simulink subsystem "EncoderAdryvelZ"  (R2023b)
settings: Solver=VariableStepAuto  StartTime=0.0  StopTime=10.0  RelTol=1e-3
libraries: arduinosensorlib x2, simulink x1
settings Model: Creator=johan  LastModifiedBy=adria

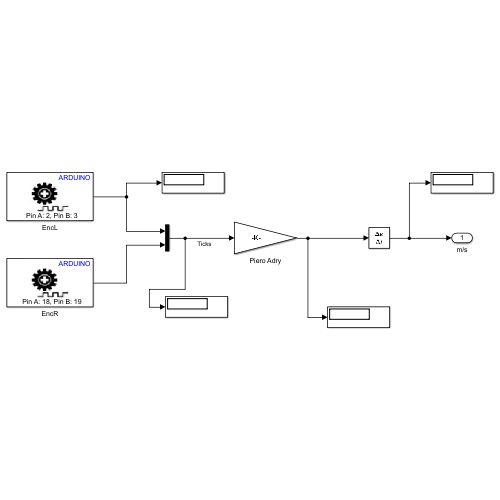
[thumbnail: Simulink's stored preview of the top-level diagram]
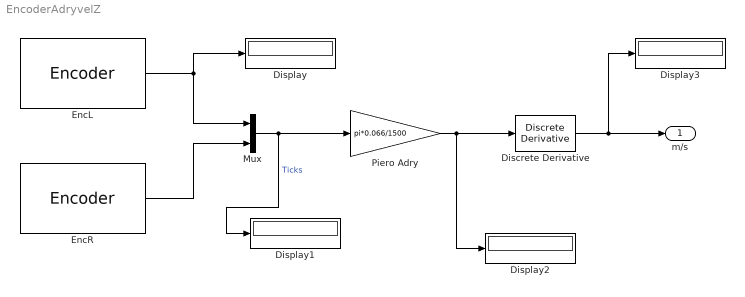
== system EncoderAdryvelZ ==
  Discrete Derivative : simulink/Discrete/Discrete Derivative  gainval=1.0  ICPrevScaledInput=0.0  OutMin=[]  OutMax=[]  OutDataType=fixdt(1, 16)  OutScaling=2^-10  DoSatur=off
  Display{,1..3} (4 alike) : Display
  EncL : arduinosensorlib/Encoder  InputA=2  InputB=3  Mode=No reset  SampleTime=-1
  EncR : arduinosensorlib/Encoder  InputA=18  InputB=19  Mode=No reset  SampleTime=-1
  Mux : Mux  Inputs=2
  Piero Adry : Gain  Gain=pi*0.066/1500  OutDataTypeStr=double
  m/s : Outport
  wires:
  EncR/1 -> Mux/2
  EncL/1 -> Mux/1, Display/1
  Mux/1 -> Piero Adry/1, Display1/1  "Ticks"
  Piero Adry/1 -> Display2/1, Discrete Derivative/1
  Discrete Derivative/1 -> m/s/1, Display3/1
